simulink model "NavFilterTestHarness21"  (Simulink 7.9)
settings: Solver=FixedStepDiscrete  StartTime=min(IMUtime)  StopTime=max(IMUtime)  FixedStep=0.001  RelTol=1e-3
undefined symbols (not defined in the file or in its folder): accel, ADSframe, ADStime, angRate, ATTframe, CourseDeg, GndSpd, GPSframe, GPStime, Hgt, IMUframe, IMUtime, LatDeg, LngDeg, MagBiasX, MagBiasY, MagBiasZ, MAGframe, MAGtime, MagX, MagY, MagZ, Pitch, Roll, Veas, VelD, Yaw
libraries: simulink x13
(part 4 of 5)

== matlab function InertialNavFilter/Fuse True Airspeed Measurements ==
  data: states input double; P input double; FuseData input double; VtasMea input double; nextStates output double; nextP output double; innovation output double; StatesAtMeasTime input double; varInnov output double; useAirspeed input double
%#codegen
function [...
    nextStates, ... % state vector after fusion of measurements
    nextP, ... % state covariance matrix after fusion of corrections
    innovation, ... % True airspeed innovations (m/s)
    varInnov] ... % True airspeed innovation variance (m/s)^2
    = FuseAirspeed( ...
    states, ... % predicted states from the INS (q0, ... , q3, VelN,E,D, PosN,E,D, WindN,E, P0, camera roll pitch yaw misalignment)
    P, ... % predicted covariance
    FuseData, ... % Boolean to initiate fusion of airspeed measurements
    VtasMea, ... % true airspeed measurement (m/s)
    StatesAtMeasTime, ... % states at time of airspeed measurement
    useAirspeed) % Boolean to indicate that a airspeed sensor is being used

% initialise innovation
innovation = single(0);

% initialise innovation variance vector (for data analysis only)
varInnov = single(0);

% Airspeed measurement error variance (m/s)^2.
R_TAS = single(2.0);

% Copy required states to local variable names
vn = single(StatesAtMeasTime(5));
ve = single(StatesAtMeasTime(6));
vd = single(StatesAtMeasTime(7));
vwn = single(StatesAtMeasTime(14));
vwe = single(StatesAtMeasTime(15));

% define arrays used to calculate intermediate result in covariance
% update
KH  = single(zeros(21,21));
KHP = single(zeros(21,21));

% Calculate the airspeed prediction
VtasPred = sqrt((ve - vwe)^2 + (vn - vwn)^2 + vd^2);
% Need to check that it is flying before fusing airspeed data due to
if (useAirspeed && FuseData && (VtasPred > 1.0) && VtasMea > 8.0)
    % Sequential fusion of XYZ components
    
    % Calculate observation jacobians and Kalman gain
    SH_TAS = single(zeros(3,1));
    SH_TAS(1) = 1/((ve - vwe)^2 + (vn - vwn)^2 + vd^2)^(1/2);
    SH_TAS(2) = (SH_TAS(1)*(2*ve - 2*vwe))/2;
    SH_TAS(3) = (SH_TAS(1)*(2*vn - 2*vwn))/2;
    
    H_TAS = single(zeros(1,21));
    H_TAS(1,5) = SH_TAS(3);
    H_TAS(1,6) = SH_TAS(2);
    H_TAS(1,7) = vd*SH_TAS(1);
    H_TAS(1,14) = -SH_TAS(3);
    H_TAS(1,15) = -SH_TAS(2);
    
    SK_TAS = single(zeros(2,1));
    SK_TAS(1) = 1/(R_TAS + SH_TAS(3)*(P(5,5)*SH_TAS(3) + P(6,5)*SH_TAS(2) - P(14,5)*SH_TAS(3) - P(15,5)*SH_TAS(2) + P(7,5)*vd*SH_TAS(1)) + SH_TAS(2)*(P(5,6)*SH_TAS(3) + P(6,6)*SH_TAS(2) - P(14,6)*SH_TAS(3) - P(15,6)*SH_TAS(2) + P(7,6)*vd*SH_TAS(1)) - SH_TAS(3)*(P(5,14)*SH_TAS(3) + P(6,14)*SH_TAS(2) - P(14,14)*SH_TAS(3) - P(15,14)*SH_TAS(2) + P(7,14)*vd*SH_TAS(1)) - SH_TAS(2)*(P(5,15)*SH_TAS(3) + P(6,15)*SH_TAS(2) - P(14,15)*SH_TAS(3) - P(15,15)*SH_TAS(2) + P(7,15)*vd*SH_TAS(1)) + vd*SH_TAS(1)*(P(5,7)*SH_TAS(3) + P(6,7)*SH_TAS(2) - P(14,7)*SH_TAS(3) - P(15,7)*SH_TAS(2) + P(7,7)*vd*SH_TAS(1)));
    SK_TAS(2) = SH_TAS(2);
    
    K_TAS = single(zeros(21,1));
    K_TAS(1,1) = SK_TAS(1)*(P(1,5)*SH_TAS(3) - P(1,14)*SH_TAS(3) + P(1,6)*SK_TAS(2) - P(1,15)*SK_TAS(2) + P(1,7)*vd*SH_TAS(1));
    K_TAS(2,1) = SK_TAS(1)*(P(2,5)*SH_TAS(3) - P(2,14)*SH_TAS(3) + P(2,6)*SK_TAS(2) - P(2,15)*SK_TAS(2) + P(2,7)*vd*SH_TAS(1));
    K_TAS(3,1) = SK_TAS(1)*(P(3,5)*SH_TAS(3) - P(3,14)*SH_TAS(3) + P(3,6)*SK_TAS(2) - P(3,15)*SK_TAS(2) + P(3,7)*vd*SH_TAS(1));
    K_TAS(4,1) = SK_TAS(1)*(P(4,5)*SH_TAS(3) - P(4,14)*SH_TAS(3) + P(4,6)*SK_TAS(2) - P(4,15)*SK_TAS(2) + P(4,7)*vd*SH_TAS(1));
    K_TAS(5,1) = SK_TAS(1)*(P(5,5)*SH_TAS(3) - P(5,14)*SH_TAS(3) + P(5,6)*SK_TAS(2) - P(5,15)*SK_TAS(2) + P(5,7)*vd*SH_TAS(1));
    K_TAS(6,1) = SK_TAS(1)*(P(6,5)*SH_TAS(3) - P(6,14)*SH_TAS(3) + P(6,6)*SK_TAS(2) - P(6,15)*SK_TAS(2) + P(6,7)*vd*SH_TAS(1));
    K_TAS(7,1) = SK_TAS(1)*(P(7,5)*SH_TAS(3) - P(7,14)*SH_TAS(3) + P(7,6)*SK_TAS(2) - P(7,15)*SK_TAS(2) + P(7,7)*vd*SH_TAS(1));
    K_TAS(8,1) = SK_TAS(1)*(P(8,5)*SH_TAS(3) - P(8,14)*SH_TAS(3) + P(8,6)*SK_TAS(2) - P(8,15)*SK_TAS(2) + P(8,7)*vd*SH_TAS(1));
    K_TAS(9,1) = SK_TAS(1)*(P(9,5)*SH_TAS(3) - P(9,14)*SH_TAS(3) + P(9,6)*SK_TAS(2) - P(9,15)*SK_TAS(2) + P(9,7)*vd*SH_TAS(1));
    K_TAS(10,1) = SK_TAS(1)*(P(10,5)*SH_TAS(3) - P(10,14)*SH_TAS(3) + P(10,6)*SK_TAS(2) - P(10,15)*SK_TAS(2) + P(10,7)*vd*SH_TAS(1));
    K_TAS(11,1) = SK_TAS(1)*(P(11,5)*SH_TAS(3) - P(11,14)*SH_TAS(3) + P(11,6)*SK_TAS(2) - P(11,15)*SK_TAS(2) + P(11,7)*vd*SH_TAS(1));
    K_TAS(12,1) = SK_TAS(1)*(P(12,5)*SH_TAS(3) - P(12,14)*SH_TAS(3) + P(12,6)*SK_TAS(2) - P(12,15)*SK_TAS(2) + P(12,7)*vd*SH_TAS(1));
    K_TAS(13,1) = SK_TAS(1)*(P(13,5)*SH_TAS(3) - P(13,14)*SH_TAS(3) + P(13,6)*SK_TAS(2) - P(13,15)*SK_TAS(2) + P(13,7)*vd*SH_TAS(1));
    K_TAS(14,1) = SK_TAS(1)*(P(14,5)*SH_TAS(3) - P(14,14)*SH_TAS(3) + P(14,6)*SK_TAS(2) - P(14,15)*SK_TAS(2) + P(14,7)*vd*SH_TAS(1));
    K_TAS(15,1) = SK_TAS(1)*(P(15,5)*SH_TAS(3) - P(15,14)*SH_TAS(3) + P(15,6)*SK_TAS(2) - P(15,15)*SK_TAS(2) + P(15,7)*vd*SH_TAS(1));
    K_TAS(16,1) = SK_TAS(1)*(P(16,5)*SH_TAS(3) - P(16,14)*SH_TAS(3) + P(16,6)*SK_TAS(2) - P(16,15)*SK_TAS(2) + P(16,7)*vd*SH_TAS(1));
    K_TAS(17,1) = SK_TAS(1)*(P(17,5)*SH_TAS(3) - P(17,14)*SH_TAS(3) + P(17,6)*SK_TAS(2) - P(17,15)*SK_TAS(2) + P(17,7)*vd*SH_TAS(1));
    K_TAS(18,1) = SK_TAS(1)*(P(18,5)*SH_TAS(3) - P(18,14)*SH_TAS(3) + P(18,6)*SK_TAS(2) - P(18,15)*SK_TAS(2) + P(18,7)*vd*SH_TAS(1));
    K_TAS(19,1) = SK_TAS(1)*(P(19,5)*SH_TAS(3) - P(19,14)*SH_TAS(3) + P(19,6)*SK_TAS(2) - P(19,15)*SK_TAS(2) + P(19,7)*vd*SH_TAS(1));
    K_TAS(20,1) = SK_TAS(1)*(P(20,5)*SH_TAS(3) - P(20,14)*SH_TAS(3) + P(20,6)*SK_TAS(2) - P(20,15)*SK_TAS(2) + P(20,7)*vd*SH_TAS(1));
    K_TAS(21,1) = SK_TAS(1)*(P(21,5)*SH_TAS(3) - P(21,14)*SH_TAS(3) + P(21,6)*SK_TAS(2) - P(21,15)*SK_TAS(2) + P(21,7)*vd*SH_TAS(1));
    
    % calculate the innovation variance (for data logging only)
    varInnov = 1/SK_TAS(1);
    
    % Calculate the measurement innovation
    innovation = VtasPred - VtasMea;
    % Check the innovation for consistencey and don't fuse if > 5Sigma
    if (innovation*innovation*SK_TAS(1)) < 25.0
        xk = K_TAS * innovation;
        states = states - xk;
        % normalise the quaternion states
        quatMag = sqrt(states(1)^2 + states(2)^2 + states(3)^2 + states(4)^2);
        if (quatMag > 1e-12)
            states(1:4) = states(1:4) / quatMag;
        end
        % correct the covariance P = (I - K*H)*P
        % take advantage of the empty columns in H_TAS to reduce the
        % number of operations
        for i = 1:24
            for j = 5:7
                KH(i,j) = K_TAS(i)*H_TAS(j);
            end
            for j = 14:15
                KH(i,j) = K_TAS(i)*H_TAS(j);
            end
        end
        for i = 1:21
            for j = 1:21
                for k = 5:7
                    KHP(i,j) = KHP(i,j) + KH(i,k)*P(k,j);
                end
                for k = 14:15
                    KHP(i,j) = KHP(i,j) + KH(i,k)*P(k,j);
                end
            end
        end
        P = P - KHP;
        P = 0.5*(P + transpose(P));
    end
end

% Set default output for states and covariance
nextP = P;
nextStates   = states;

end

== matlab function InertialNavFilter/Store States at Magnetometer Meas Time ==
  data: FuseData output double; States input double; measDataArrived input double; StatesAtMeasTime output double; Ndelay input double; ratio input double
%#codegen
function [FuseData,StatesAtMeasTime]   = StoreStatesAtMeasTime(States,measDataArrived,Ndelay,ratio)

% Implement a state sampler that stores the state inoput from Ndelay 
% samples before the measurement is predicted to arrive. When the
% measurement arrives, the stored state is output along with a data fusion
% request. This enables the filter to account for lag in sensors that can
% in some cases be greater than 1 measurement time step. the delay time si
% specified in units of the state prediction delta time. For example if a 
% delay of 0.16 seconds was required, and the state prediction ran at 50 Hz
% then Ndelay would be set to 50*0.15 = 8.
% It is assumed that this function is called the same rate as the state 
% prediction, and that the measurement data comes in at a constant
% rate.
% The 'ratio'specifies the ratio of the state prediction to measurement
% data rates. For example if the state prediction occurres at 50Hz and the
% measurements are being received at 5Hz, then 'ratio' = 50/5 = 10

% This function avoids the need to use large data buffers
% It is generic function that can be used for states required by all
% measurement fusion processes, and as such has not been optimised to only
% includes the specific states required, or the buffer arry length trimmed
% to the minimum required.

% Ndelay cannot be zero and cannot exceed a value of 10*ratio-1
Ndelay = max(min(Ndelay,int32(10*ratio)),int32(1));

majorStepDelay = int32(ceil(single(Ndelay)/single(ratio)));
minorStepDelay = int32(rem(single(Ndelay),single(ratio)));

persistent prevStatesMatrix;
if isempty(prevStatesMatrix)
    prevStatesMatrix = single(zeros(21,11));
end

persistent totalFrameCount;
if isempty(totalFrameCount)
    totalFrameCount = int32(0);
end

persistent measID;
if isempty(measID)
    measID = int32(zeros(1,11));
end

persistent minorFrameCount;
if isempty(minorFrameCount)
    minorFrameCount = int32(0);
end

totalFrameCount = totalFrameCount + int32(1);
minorFrameCount = minorFrameCount + int32(1);

if measDataArrived
    if measID(1) ~= 0
        FuseData = logical(1);
    else
        FuseData = logical(0);
    end
    if abs(single(totalFrameCount - measID(1) - Ndelay)) < 0.5*single(ratio)
        StatesAtMeasTime = prevStatesMatrix(:,1);
    else
        frameErrors = abs(measID - totalFrameCount + Ndelay);
        bestError = Ndelay;
        bestIndex = int32(1);
        for index = 1:majorStepDelay
            if frameErrors(index) < bestError
                bestError = frameErrors(index);
                bestIndex = index;
            end
        end
        StatesAtMeasTime = prevStatesMatrix(:,bestIndex);
    end
else
    StatesAtMeasTime = single(zeros(21,1));
    FuseData = logical(0);
end

if minorFrameCount == (ratio - minorStepDelay)
    if majorStepDelay > int32(0)
        for index = 1:majorStepDelay
            prevStatesMatrix(:,index) = prevStatesMatrix(:,index+1);
            measID(index) = measID(index+1);
        end
    end
    prevStatesMatrix(:,majorStepDelay) = States;
    measID(majorStepDelay) = totalFrameCount;
end

if measDataArrived
    minorFrameCount = int32(0);
end

end

== matlab function InertialNavFilter/Calc Initial Parameters/Embedded MATLAB Function ==
  data: gravityNED output double; earthRateNED output double; covariance output double; latDeg input double
function [gravityNED, earthRateNED, covariance] = calculateInitialData(latDeg)
%#codegen

% degrees to to radians conversion
deg2rad = single(pi/180);

% Define the local gracity vector
gravityNED  = single([0;0;9.807]);

% Define the initial Euler angle covariance (Phi, Theta, Psi)
InitialEulerCovariance  = single([(1.0*pi/180); (1.0*pi/180); (10.0*pi/180)].^2);

% Define the transformation vector from a 321 sequence Euler rotation vector to a q0,...,q3 quaternion vector
% linearised around a level orientation (roll,pitch = 0,0)
J_eul2quat = ...
    single([[ 0.0, 0.0, 0.0]; ...
    [ 0.5, 0.0, 0.0]; ...
    [ 0.0, 0.5, 0.0]; ...
    [ 0.0, 0.0, 0.5]]);

% Form the covariance matrix for the intial Euler angle coordinates
angleCov = diag(InitialEulerCovariance);

% Transform the Euler angle covariances into the equivalent quaternion covariances
quatCov = J_eul2quat*angleCov*transpose(J_eul2quat);

% define the state covariances with the exception of the quaternion covariances
Sigma_vel_NE = single(0.7); % 1 sigma uncertainty in horizontal velocity components
Sigma_vel_D  = single(0.7); % 1 sigma uncertainty in vertical velocity
Sigma_pos_NE = single(15); % 1 sigma uncertainty in horizontal position components
Sigma_pos_D  = single(5.0); % 1 sigma uncertainty in vertical position
Sigma_dAng   = single(1/10*pi/180*0.02); % 1 Sigma uncertainty in delta angle bias
Sigma_wind   = single(8);
Sigma_MagNED = single(20);
Sigma_MagXYZ = single(20);
covariance   = single(diag([0;0;0;0;Sigma_vel_NE*[1;1];Sigma_vel_D;Sigma_pos_NE*[1;1];Sigma_pos_D;Sigma_dAng*[1;1;1];Sigma_wind*[1;1];Sigma_MagNED*[1;1;1];Sigma_MagXYZ*[1;1;1]].^2));

% Add the quaternion covariances
covariance(1:4,1:4) = quatCov;

%Define Earth rotation vector in the NED navigation frame
earthRateECEF = single([0; 0; 7.2921e-005]);
earthRateNED  = ...
    single([cos(latDeg*deg2rad)*earthRateECEF(3); ...
    0; ...
    -sin(latDeg*deg2rad)*earthRateECEF(3)]);

== matlab function InertialNavFilter/Store States at Height Meas Time ==
  data: FuseData output double; States input double; measDataArrived input double; StatesAtMeasTime output double; Ndelay input double; ratio input double
%#codegen
function [FuseData,StatesAtMeasTime]   = StoreStatesAtMeasTime(States,measDataArrived,Ndelay,ratio)

% Implement a state sampler that stores the state inoput from Ndelay 
% samples before the measurement is predicted to arrive. When the
% measurement arrives, the stored state is output along with a data fusion
% request. This enables the filter to account for lag in sensors that can
% in some cases be greater than 1 measurement time step. the delay time si
% specified in units of the state prediction delta time. For example if a 
% delay of 0.16 seconds was required, and the state prediction ran at 50 Hz
% then Ndelay would be set to 50*0.15 = 8.
% It is assumed that this function is called the same rate as the state 
% prediction, and that the measurement data comes in at a constant
% rate.
% The 'ratio'specifies the ratio of the state prediction to measurement
% data rates. For example if the state prediction occurres at 50Hz and the
% measurements are being received at 5Hz, then 'ratio' = 50/5 = 10

% This function avoids the need to use large data buffers
% It is generic function that can be used for states required by all
% measurement fusion processes, and as such has not been optimised to only
% includes the specific states required, or the buffer arry length trimmed
% to the minimum required.

% Ndelay cannot be zero and cannot exceed a value of 10*ratio-1
Ndelay = max(min(Ndelay,int32(10*ratio)),int32(1));

majorStepDelay = int32(ceil(single(Ndelay)/single(ratio)));
minorStepDelay = int32(rem(single(Ndelay),single(ratio)));

persistent prevStatesMatrix;
if isempty(prevStatesMatrix)
    prevStatesMatrix = single(zeros(21,11));
end

persistent totalFrameCount;
if isempty(totalFrameCount)
    totalFrameCount = int32(0);
end

persistent measID;
if isempty(measID)
    measID = int32(zeros(1,11));
end

persistent minorFrameCount;
if isempty(minorFrameCount)
    minorFrameCount = int32(0);
end

totalFrameCount = totalFrameCount + int32(1);
minorFrameCount = minorFrameCount + int32(1);

if measDataArrived
    if measID(1) ~= 0
        FuseData = logical(1);
    else
        FuseData = logical(0);
    end
    if abs(single(totalFrameCount - measID(1) - Ndelay)) < 0.5*single(ratio)
        StatesAtMeasTime = prevStatesMatrix(:,1);
    else
        frameErrors = abs(measID - totalFrameCount + Ndelay);
        bestError = Ndelay;
        bestIndex = int32(1);
        for index = 1:majorStepDelay
            if frameErrors(index) < bestError
                bestError = frameErrors(index);
                bestIndex = index;
            end
        end
        StatesAtMeasTime = prevStatesMatrix(:,bestIndex);
    end
else
    StatesAtMeasTime = single(zeros(21,1));
    FuseData = logical(0);
end

if minorFrameCount == (ratio - minorStepDelay)
    if majorStepDelay > int32(0)
        for index = 1:majorStepDelay
            prevStatesMatrix(:,index) = prevStatesMatrix(:,index+1);
            measID(index) = measID(index+1);
        end
    end
    prevStatesMatrix(:,majorStepDelay) = States;
    measID(majorStepDelay) = totalFrameCount;
end

if measDataArrived
    minorFrameCount = int32(0);
end

end

== matlab function InertialNavFilter/Store States at Vtas Meas Time ==
  data: FuseData output double; States input double; measDataArrived input double; StatesAtMeasTime output double; Ndelay input double; ratio input double
%#codegen
function [FuseData,StatesAtMeasTime]   = StoreStatesAtMeasTime(States,measDataArrived,Ndelay,ratio)

% Implement a state sampler that stores the state inoput from Ndelay 
% samples before the measurement is predicted to arrive. When the
% measurement arrives, the stored state is output along with a data fusion
% request. This enables the filter to account for lag in sensors that can
% in some cases be greater than 1 measurement time step. the delay time si
% specified in units of the state prediction delta time. For example if a 
% delay of 0.16 seconds was required, and the state prediction ran at 50 Hz
% then Ndelay would be set to 50*0.15 = 8.
% It is assumed that this function is called the same rate as the state 
% prediction, and that the measurement data comes in at a constant
% rate.
% The 'ratio'specifies the ratio of the state prediction to measurement
% data rates. For example if the state prediction occurres at 50Hz and the
% measurements are being received at 5Hz, then 'ratio' = 50/5 = 10

% This function avoids the need to use large data buffers
% It is generic function that can be used for states required by all
% measurement fusion processes, and as such has not been optimised to only
% includes the specific states required, or the buffer arry length trimmed
% to the minimum required.

% Ndelay cannot be zero and cannot exceed a value of 10*ratio-1
Ndelay = max(min(Ndelay,int32(10*ratio)),int32(1));

majorStepDelay = int32(ceil(single(Ndelay)/single(ratio)));
minorStepDelay = int32(rem(single(Ndelay),single(ratio)));

persistent prevStatesMatrix;
if isempty(prevStatesMatrix)
    prevStatesMatrix = single(zeros(21,11));
end

persistent totalFrameCount;
if isempty(totalFrameCount)
    totalFrameCount = int32(0);
end

persistent measID;
if isempty(measID)
    measID = int32(zeros(1,11));
end

persistent minorFrameCount;
if isempty(minorFrameCount)
    minorFrameCount = int32(0);
end

totalFrameCount = totalFrameCount + int32(1);
minorFrameCount = minorFrameCount + int32(1);

if measDataArrived
    if measID(1) ~= 0
        FuseData = logical(1);
    else
        FuseData = logical(0);
    end
    if abs(single(totalFrameCount - measID(1) - Ndelay)) < 0.5*single(ratio)
        StatesAtMeasTime = prevStatesMatrix(:,1);
    else
        frameErrors = abs(measID - totalFrameCount + Ndelay);
        bestError = Ndelay;
        bestIndex = int32(1);
        for index = 1:majorStepDelay
            if frameErrors(index) < bestError
                bestError = frameErrors(index);
                bestIndex = index;
            end
        end
        StatesAtMeasTime = prevStatesMatrix(:,bestIndex);
    end
else
    StatesAtMeasTime = single(zeros(21,1));
    FuseData = logical(0);
end

if minorFrameCount == (ratio - minorStepDelay)
    if majorStepDelay > int32(0)
        for index = 1:majorStepDelay
            prevStatesMatrix(:,index) = prevStatesMatrix(:,index+1);
            measID(index) = measID(index+1);
        end
    end
    prevStatesMatrix(:,majorStepDelay) = States;
    measID(majorStepDelay) = totalFrameCount;
end

if measDataArrived
    minorFrameCount = int32(0);
end

end

== matlab function InertialNavFilter/Fuse Magnetometer Measurements ==
  data: states input double; P input double; FuseData input double; MagData input double; StatesAtMeasTime input double; nextStates output double; nextP output double; innovation output double; varInnov output double; useCompass input double
%#codegen
function [...
    nextStates, ... % state vector after fusion of measurements
    nextP, ... % state covariance matrix after fusion of corrections
    innovation, ... % Magnetometer innovations - milligauss
    varInnov] ... % Innovation variances - millgauss^2
    = FuseMagnetometer( ...
    states, ... % predicted states
    P, ... % predicted covariance
    FuseData, ... % Boolean to initiate fusion of magnetometer measurements
    MagData, ... % Magnetic flux measurements (milliGauss)
    StatesAtMeasTime, ... % states at time of airspeed measurement
    useCompass) % Boolean to indicate that a Magnetometer is being used

persistent q0 q1 q2 q3 magN magE magD;
if isempty(q0)
    q0 = single(1);
end
if isempty(q1)
    q1 = single(0);
end
if isempty(q2)
    q2 = single(0);
end
if isempty(q3)
    q3 = single(0);
end
if isempty(magN)
    magN = single(0);
end
if isempty(magE)
    magE = single(0);
end
if isempty(magD)
    magD = single(0);
end
persistent obsIndex
if isempty(obsIndex)
    obsIndex = 1;
end
persistent SH_MAG
if isempty(SH_MAG)
    SH_MAG = single(zeros(9,1));
end
persistent Tnb
if isempty(Tnb)
    Tnb = single(eye(3,3));
end
persistent MagPred
if isempty(MagPred)
    MagPred = single(zeros(3,1));
end

% declare array used to calculate intermediate result in covariance
% update
KH  = single(zeros(21,21));
KHP = single(zeros(21,21));

% define magnetometer measurement error variance (milligauss).
R_MAG = single(50^2);

% declare innovation variances
varInnov = single(zeros(3,1));

% declare innovation vector
innovation = single(zeros(1,3));

% Perform sequential fusion of Magnetometer measurements.
% This assumes that the errors in the dfferent componenets are
% uncorrelated which is not true, however in the absence of covariance
% data fit is the only assumption we can make
% so we might as well take advantage of the computational efficiencies
% associated with sequential fusion
if (useCompass && FuseData) || (useCompass && (obsIndex == 2 || obsIndex == 3))
    % Sequential fusion of XYZ components to spread processing load across
    % three prediction time steps.
    % Calculate observation jacobians and Kalman gains
    K_MAG = single(zeros(21,1));
    H_MAG = single(zeros(1,21));
    if FuseData
        % Copy required states to local variable names
        q0 = StatesAtMeasTime(1);
        q1 = StatesAtMeasTime(2);
        q2 = StatesAtMeasTime(3);
        q3 = StatesAtMeasTime(4);
        magN = StatesAtMeasTime(16);
        magE = StatesAtMeasTime(17);
        magD = StatesAtMeasTime(18);
        % rotate predicted earth components into body axes and calculate
        % predicted measurments
        Tnb = single([q0^2 + q1^2 - q2^2 - q3^2, 2*(q1*q2 + q0*q3) , 2*(q1*q3-q0*q2) ;...
            2*(q1*q2 - q0*q3), q0^2 - q1^2 + q2^2 - q3^2, 2*(q2*q3 + q0*q1);...
            2*(q1*q3 + q0*q2) , 2*(q2*q3 - q0*q1) , q0^2 - q1^2 - q2^2 + q3^2]);
        MagPred = Tnb*StatesAtMeasTime(16:18) + StatesAtMeasTime(19:21);
        % Calculate observation jacobian common terms
        SH_MAG(1) = 2*magD*q3 + 2*magE*q2 + 2*magN*q1;
        SH_MAG(2) = 2*magD*q0 - 2*magE*q1 + 2*magN*q2;
        SH_MAG(3) = 2*magD*q1 + 2*magE*q0 - 2*magN*q3;
        SH_MAG(4) = q3^2;
        SH_MAG(5) = q2^2;
        SH_MAG(6) = q1^2;
        SH_MAG(7) = q0^2;
        SH_MAG(8) = 2*magN*q0;
        SH_MAG(9) = 2*magE*q3;
        % calculate observation jacobian
        H_MAG = single(zeros(1,21));
        H_MAG(1,1) = SH_MAG(8) + SH_MAG(9) - 2*magD*q2;
        H_MAG(1,2) = SH_MAG(1);
        H_MAG(1,3) = 2*magE*q1 - 2*magD*q0 - 2*magN*q2;
        H_MAG(1,4) = SH_MAG(3);
        H_MAG(1,16) = SH_MAG(6) - SH_MAG(5) - SH_MAG(4) + SH_MAG(7);
        H_MAG(1,17) = 2*q0*q3 + 2*q1*q2;
        H_MAG(1,18) = 2*q1*q3 - 2*q0*q2;
        H_MAG(1,19) = 1;
        % calculate Kalman gain
        SK_MX = zeros(6,1);
        SK_MX(1) = 1/(P(19,19) + R_MAG + P(2,19)*SH_MAG(1) + P(4,19)*SH_MAG(3) - P(16,19)*(SH_MAG(4) + SH_MAG(5) - SH_MAG(6) - SH_MAG(7)) - (2*magD*q0 - 2*magE*q1 + 2*magN*q2)*(P(19,3) + P(2,3)*SH_MAG(1) + P(4,3)*SH_MAG(3) - P(16,3)*(SH_MAG(4) + SH_MAG(5) - SH_MAG(6) - SH_MAG(7)) + P(17,3)*(2*q0*q3 + 2*q1*q2) - P(18,3)*(2*q0*q2 - 2*q1*q3) - P(3,3)*(2*magD*q0 - 2*magE*q1 + 2*magN*q2) + P(1,3)*(SH_MAG(8) + SH_MAG(9) - 2*magD*q2)) + (SH_MAG(8) + SH_MAG(9) - 2*magD*q2)*(P(19,1) + P(2,1)*SH_MAG(1) + P(4,1)*SH_MAG(3) - P(16,1)*(SH_MAG(4) + SH_MAG(5) - SH_MAG(6) - SH_MAG(7)) + P(17,1)*(2*q0*q3 + 2*q1*q2) - P(18,1)*(2*q0*q2 - 2*q1*q3) - P(3,1)*(2*magD*q0 - 2*magE*q1 + 2*magN*q2) + P(1,1)*(SH_MAG(8) + SH_MAG(9) - 2*magD*q2)) + SH_MAG(1)*(P(19,2) + P(2,2)*SH_MAG(1) + P(4,2)*SH_MAG(3) - P(16,2)*(SH_MAG(4) + SH_MAG(5) - SH_MAG(6) - SH_MAG(7)) + P(17,2)*(2*q0*q3 + 2*q1*q2) - P(18,2)*(2*q0*q2 - 2*q1*q3) - P(3,2)*(2*magD*q0 - 2*magE*q1 + 2*magN*q2) + P(1,2)*(SH_MAG(8) + SH_MAG(9) - 2*magD*q2)) + SH_MAG(3)*(P(19,4) + P(2,4)*SH_MAG(1) + P(4,4)*SH_MAG(3) - P(16,4)*(SH_MAG(4) + SH_MAG(5) - SH_MAG(6) - SH_MAG(7)) + P(17,4)*(2*q0*q3 + 2*q1*q2) - P(18,4)*(2*q0*q2 - 2*q1*q3) - P(3,4)*(2*magD*q0 - 2*magE*q1 + 2*magN*q2) + P(1,4)*(SH_MAG(8) + SH_MAG(9) - 2*magD*q2)) - (SH_MAG(4) + SH_MAG(5) - SH_MAG(6) - SH_MAG(7))*(P(19,16) + P(2,16)*SH_MAG(1) + P(4,16)*SH_MAG(3) - P(16,16)*(SH_MAG(4) + SH_MAG(5) - SH_MAG(6) - SH_MAG(7)) + P(17,16)*(2*q0*q3 + 2*q1*q2) - P(18,16)*(2*q0*q2 - 2*q1*q3) - P(3,16)*(2*magD*q0 - 2*magE*q1 + 2*magN*q2) + P(1,16)*(SH_MAG(8) + SH_MAG(9) - 2*magD*q2)) + P(17,19)*(2*q0*q3 + 2*q1*q2) - P(18,19)*(2*q0*q2 - 2*q1*q3) - P(3,19)*(2*magD*q0 - 2*magE*q1 + 2*magN*q2) + (2*q0*q3 + 2*q1*q2)*(P(19,17) + P(2,17)*SH_MAG(1) + P(4,17)*SH_MAG(3) - P(16,17)*(SH_MAG(4) + SH_MAG(5) - SH_MAG(6) - SH_MAG(7)) + P(17,17)*(2*q0*q3 + 2*q1*q2) - P(18,17)*(2*q0*q2 - 2*q1*q3) - P(3,17)*(2*magD*q0 - 2*magE*q1 + 2*magN*q2) + P(1,17)*(SH_MAG(8) + SH_MAG(9) - 2*magD*q2)) - (2*q0*q2 - 2*q1*q3)*(P(19,18) + P(2,18)*SH_MAG(1) + P(4,18)*SH_MAG(3) - P(16,18)*(SH_MAG(4) + SH_MAG(5) - SH_MAG(6) - SH_MAG(7)) + P(17,18)*(2*q0*q3 + 2*q1*q2) - P(18,18)*(2*q0*q2 - 2*q1*q3) - P(3,18)*(2*magD*q0 - 2*magE*q1 + 2*magN*q2) + P(1,18)*(SH_MAG(8) + SH_MAG(9) - 2*magD*q2)) + P(1,19)*(SH_MAG(8) + SH_MAG(9) - 2*magD*q2));
        SK_MX(2) = SH_MAG(4) + SH_MAG(5) - SH_MAG(6) - SH_MAG(7);
        SK_MX(3) = 2*magD*q0 - 2*magE*q1 + 2*magN*q2;
        SK_MX(4) = SH_MAG(8) + SH_MAG(9) - 2*magD*q2;
        SK_MX(5) = 2*q0*q2 - 2*q1*q3;
        SK_MX(6) = 2*q0*q3 + 2*q1*q2;
        K_MAG = single(zeros(21,1));
        K_MAG(1,1) = SK_MX(1)*(P(1,19) + P(1,2)*SH_MAG(1) + P(1,4)*SH_MAG(3) + P(1,1)*SK_MX(4) - P(1,3)*SK_MX(3) - P(1,16)*SK_MX(2) + P(1,17)*SK_MX(6) - P(1,18)*SK_MX(5));
        K_MAG(2,1) = SK_MX(1)*(P(2,19) + P(2,2)*SH_MAG(1) + P(2,4)*SH_MAG(3) + P(2,1)*SK_MX(4) - P(2,3)*SK_MX(3) - P(2,16)*SK_MX(2) + P(2,17)*SK_MX(6) - P(2,18)*SK_MX(5));
        K_MAG(3,1) = SK_MX(1)*(P(3,19) + P(3,2)*SH_MAG(1) + P(3,4)*SH_MAG(3) + P(3,1)*SK_MX(4) - P(3,3)*SK_MX(3) - P(3,16)*SK_MX(2) + P(3,17)*SK_MX(6) - P(3,18)*SK_MX(5));
        K_MAG(4,1) = SK_MX(1)*(P(4,19) + P(4,2)*SH_MAG(1) + P(4,4)*SH_MAG(3) + P(4,1)*SK_MX(4) - P(4,3)*SK_MX(3) - P(4,16)*SK_MX(2) + P(4,17)*SK_MX(6) - P(4,18)*SK_MX(5));
        K_MAG(5,1) = SK_MX(1)*(P(5,19) + P(5,2)*SH_MAG(1) + P(5,4)*SH_MAG(3) + P(5,1)*SK_MX(4) - P(5,3)*SK_MX(3) - P(5,16)*SK_MX(2) + P(5,17)*SK_MX(6) - P(5,18)*SK_MX(5));
        K_MAG(6,1) = SK_MX(1)*(P(6,19) + P(6,2)*SH_MAG(1) + P(6,4)*SH_MAG(3) + P(6,1)*SK_MX(4) - P(6,3)*SK_MX(3) - P(6,16)*SK_MX(2) + P(6,17)*SK_MX(6) - P(6,18)*SK_MX(5));
        K_MAG(7,1) = SK_MX(1)*(P(7,19) + P(7,2)*SH_MAG(1) + P(7,4)*SH_MAG(3) + P(7,1)*SK_MX(4) - P(7,3)*SK_MX(3) - P(7,16)*SK_MX(2) + P(7,17)*SK_MX(6) - P(7,18)*SK_MX(5));
        K_MAG(8,1) = SK_MX(1)*(P(8,19) + P(8,2)*SH_MAG(1) + P(8,4)*SH_MAG(3) + P(8,1)*SK_MX(4) - P(8,3)*SK_MX(3) - P(8,16)*SK_MX(2) + P(8,17)*SK_MX(6) - P(8,18)*SK_MX(5));
        K_MAG(9,1) = SK_MX(1)*(P(9,19) + P(9,2)*SH_MAG(1) + P(9,4)*SH_MAG(3) + P(9,1)*SK_MX(4) - P(9,3)*SK_MX(3) - P(9,16)*SK_MX(2) + P(9,17)*SK_MX(6) - P(9,18)*SK_MX(5));
        K_MAG(10,1) = SK_MX(1)*(P(10,19) + P(10,2)*SH_MAG(1) + P(10,4)*SH_MAG(3) + P(10,1)*SK_MX(4) - P(10,3)*SK_MX(3) - P(10,16)*SK_MX(2) + P(10,17)*SK_MX(6) - P(10,18)*SK_MX(5));
        K_MAG(11,1) = SK_MX(1)*(P(11,19) + P(11,2)*SH_MAG(1) + P(11,4)*SH_MAG(3) + P(11,1)*SK_MX(4) - P(11,3)*SK_MX(3) - P(11,16)*SK_MX(2) + P(11,17)*SK_MX(6) - P(11,18)*SK_MX(5));
        K_MAG(12,1) = SK_MX(1)*(P(12,19) + P(12,2)*SH_MAG(1) + P(12,4)*SH_MAG(3) + P(12,1)*SK_MX(4) - P(12,3)*SK_MX(3) - P(12,16)*SK_MX(2) + P(12,17)*SK_MX(6) - P(12,18)*SK_MX(5));
        K_MAG(13,1) = SK_MX(1)*(P(13,19) + P(13,2)*SH_MAG(1) + P(13,4)*SH_MAG(3) + P(13,1)*SK_MX(4) - P(13,3)*SK_MX(3) - P(13,16)*SK_MX(2) + P(13,17)*SK_MX(6) - P(13,18)*SK_MX(5));
        K_MAG(14,1) = SK_MX(1)*(P(14,19) + P(14,2)*SH_MAG(1) + P(14,4)*SH_MAG(3) + P(14,1)*SK_MX(4) - P(14,3)*SK_MX(3) - P(14,16)*SK_MX(2) + P(14,17)*SK_MX(6) - P(14,18)*SK_MX(5));
        K_MAG(15,1) = SK_MX(1)*(P(15,19) + P(15,2)*SH_MAG(1) + P(15,4)*SH_MAG(3) + P(15,1)*SK_MX(4) - P(15,3)*SK_MX(3) - P(15,16)*SK_MX(2) + P(15,17)*SK_MX(6) - P(15,18)*SK_MX(5));
        K_MAG(16,1) = SK_MX(1)*(P(16,19) + P(16,2)*SH_MAG(1) + P(16,4)*SH_MAG(3) + P(16,1)*SK_MX(4) - P(16,3)*SK_MX(3) - P(16,16)*SK_MX(2) + P(16,17)*SK_MX(6) - P(16,18)*SK_MX(5));
        K_MAG(17,1) = SK_MX(1)*(P(17,19) + P(17,2)*SH_MAG(1) + P(17,4)*SH_MAG(3) + P(17,1)*SK_MX(4) - P(17,3)*SK_MX(3) - P(17,16)*SK_MX(2) + P(17,17)*SK_MX(6) - P(17,18)*SK_MX(5));
        K_MAG(18,1) = SK_MX(1)*(P(18,19) + P(18,2)*SH_MAG(1) + P(18,4)*SH_MAG(3) + P(18,1)*SK_MX(4) - P(18,3)*SK_MX(3) - P(18,16)*SK_MX(2) + P(18,17)*SK_MX(6) - P(18,18)*SK_MX(5));
        K_MAG(19,1) = SK_MX(1)*(P(19,19) + P(19,2)*SH_MAG(1) + P(19,4)*SH_MAG(3) + P(19,1)*SK_MX(4) - P(19,3)*SK_MX(3) - P(19,16)*SK_MX(2) + P(19,17)*SK_MX(6) - P(19,18)*SK_MX(5));
        K_MAG(20,1) = SK_MX(1)*(P(20,19) + P(20,2)*SH_MAG(1) + P(20,4)*SH_MAG(3) + P(20,1)*SK_MX(4) - P(20,3)*SK_MX(3) - P(20,16)*SK_MX(2) + P(20,17)*SK_MX(6) - P(20,18)*SK_MX(5));
        K_MAG(21,1) = SK_MX(1)*(P(21,19) + P(21,2)*SH_MAG(1) + P(21,4)*SH_MAG(3) + P(21,1)*SK_MX(4) - P(21,3)*SK_MX(3) - P(21,16)*SK_MX(2) + P(21,17)*SK_MX(6) - P(21,18)*SK_MX(5));
        varInnov(1) = 1/SK_MX(1);
        % reset the observation index to 1 (we start by fusing the X
        % measurement)
        obsIndex = 1;
    elseif obsIndex == 2 % we are now fusing the Y measurement
        H_MAG = single(zeros(1,21));
        H_MAG(1,1) = SH_MAG(3);
        H_MAG(1,2) = SH_MAG(2);
        H_MAG(1,3) = SH_MAG(1);
        H_MAG(1,4) = 2*magD*q2 - SH_MAG(9) - SH_MAG(8);
        H_MAG(1,16) = 2*q1*q2 - 2*q0*q3;
        H_MAG(1,17) = SH_MAG(5) - SH_MAG(4) - SH_MAG(6) + SH_MAG(7);
        H_MAG(1,18) = 2*q0*q1 + 2*q2*q3;
        H_MAG(1,20) = 1;
        % calculate the Kalman gain
        SK_MY = single(zeros(5,1));
        SK_MY(1) = 1/(P(20,20) + R_MAG + P(1,20)*SH_MAG(3) + P(2,20)*SH_MAG(2) + P(3,20)*SH_MAG(1) - P(17,20)*(SH_MAG(4) - SH_MAG(5) + SH_MAG(6) - SH_MAG(7)) - (2*q0*q3 - 2*q1*q2)*(P(20,16) + P(1,16)*SH_MAG(3) + P(2,16)*SH_MAG(2) + P(3,16)*SH_MAG(1) - P(17,16)*(SH_MAG(4) - SH_MAG(5) + SH_MAG(6) - SH_MAG(7)) - P(16,16)*(2*q0*q3 - 2*q1*q2) + P(18,16)*(2*q0*q1 + 2*q2*q3) - P(4,16)*(SH_MAG(8) + SH_MAG(9) - 2*magD*q2)) + (2*q0*q1 + 2*q2*q3)*(P(20,18) + P(1,18)*SH_MAG(3) + P(2,18)*SH_MAG(2) + P(3,18)*SH_MAG(1) - P(17,18)*(SH_MAG(4) - SH_MAG(5) + SH_MAG(6) - SH_MAG(7)) - P(16,18)*(2*q0*q3 - 2*q1*q2) + P(18,18)*(2*q0*q1 + 2*q2*q3) - P(4,18)*(SH_MAG(8) + SH_MAG(9) - 2*magD*q2)) - (SH_MAG(8) + SH_MAG(9) - 2*magD*q2)*(P(20,4) + P(1,4)*SH_MAG(3) + P(2,4)*SH_MAG(2) + P(3,4)*SH_MAG(1) - P(17,4)*(SH_MAG(4) - SH_MAG(5) + SH_MAG(6) - SH_MAG(7)) - P(16,4)*(2*q0*q3 - 2*q1*q2) + P(18,4)*(2*q0*q1 + 2*q2*q3) - P(4,4)*(SH_MAG(8) + SH_MAG(9) - 2*magD*q2)) - P(16,20)*(2*q0*q3 - 2*q1*q2) + P(18,20)*(2*q0*q1 + 2*q2*q3) + SH_MAG(3)*(P(20,1) + P(1,1)*SH_MAG(3) + P(2,1)*SH_MAG(2) + P(3,1)*SH_MAG(1) - P(17,1)*(SH_MAG(4) - SH_MAG(5) + SH_MAG(6) - SH_MAG(7)) - P(16,1)*(2*q0*q3 - 2*q1*q2) + P(18,1)*(2*q0*q1 + 2*q2*q3) - P(4,1)*(SH_MAG(8) + SH_MAG(9) - 2*magD*q2)) + SH_MAG(2)*(P(20,2) + P(1,2)*SH_MAG(3) + P(2,2)*SH_MAG(2) + P(3,2)*SH_MAG(1) - P(17,2)*(SH_MAG(4) - SH_MAG(5) + SH_MAG(6) - SH_MAG(7)) - P(16,2)*(2*q0*q3 - 2*q1*q2) + P(18,2)*(2*q0*q1 + 2*q2*q3) - P(4,2)*(SH_MAG(8) + SH_MAG(9) - 2*magD*q2)) + SH_MAG(1)*(P(20,3) + P(1,3)*SH_MAG(3) + P(2,3)*SH_MAG(2) + P(3,3)*SH_MAG(1) - P(17,3)*(SH_MAG(4) - SH_MAG(5) + SH_MAG(6) - SH_MAG(7)) - P(16,3)*(2*q0*q3 - 2*q1*q2) + P(18,3)*(2*q0*q1 + 2*q2*q3) - P(4,3)*(SH_MAG(8) + SH_MAG(9) - 2*magD*q2)) - (SH_MAG(4) - SH_MAG(5) + SH_MAG(6) - SH_MAG(7))*(P(20,17) + P(1,17)*SH_MAG(3) + P(2,17)*SH_MAG(2) + P(3,17)*SH_MAG(1) - P(17,17)*(SH_MAG(4) - SH_MAG(5) + SH_MAG(6) - SH_MAG(7)) - P(16,17)*(2*q0*q3 - 2*q1*q2) + P(18,17)*(2*q0*q1 + 2*q2*q3) - P(4,17)*(SH_MAG(8) + SH_MAG(9) - 2*magD*q2)) - P(4,20)*(SH_MAG(8) + SH_MAG(9) - 2*magD*q2));
        SK_MY(2) = SH_MAG(4) - SH_MAG(5) + SH_MAG(6) - SH_MAG(7);
        SK_MY(3) = SH_MAG(8) + SH_MAG(9) - 2*magD*q2;
        SK_MY(4) = 2*q0*q3 - 2*q1*q2;
        SK_MY(5) = 2*q0*q1 + 2*q2*q3;
        K_MAG = single(zeros(21,1));
        K_MAG(1,1) = SK_MY(1)*(P(1,20) + P(1,1)*SH_MAG(3) + P(1,2)*SH_MAG(2) + P(1,3)*SH_MAG(1) - P(1,4)*SK_MY(3) - P(1,17)*SK_MY(2) - P(1,16)*SK_MY(4) + P(1,18)*SK_MY(5));
        K_MAG(2,1) = SK_MY(1)*(P(2,20) + P(2,1)*SH_MAG(3) + P(2,2)*SH_MAG(2) + P(2,3)*SH_MAG(1) - P(2,4)*SK_MY(3) - P(2,17)*SK_MY(2) - P(2,16)*SK_MY(4) + P(2,18)*SK_MY(5));
        K_MAG(3,1) = SK_MY(1)*(P(3,20) + P(3,1)*SH_MAG(3) + P(3,2)*SH_MAG(2) + P(3,3)*SH_MAG(1) - P(3,4)*SK_MY(3) - P(3,17)*SK_MY(2) - P(3,16)*SK_MY(4) + P(3,18)*SK_MY(5));
        K_MAG(4,1) = SK_MY(1)*(P(4,20) + P(4,1)*SH_MAG(3) + P(4,2)*SH_MAG(2) + P(4,3)*SH_MAG(1) - P(4,4)*SK_MY(3) - P(4,17)*SK_MY(2) - P(4,16)*SK_MY(4) + P(4,18)*SK_MY(5));
        K_MAG(5,1) = SK_MY(1)*(P(5,20) + P(5,1)*SH_MAG(3) + P(5,2)*SH_MAG(2) + P(5,3)*SH_MAG(1) - P(5,4)*SK_MY(3) - P(5,17)*SK_MY(2) - P(5,16)*SK_MY(4) + P(5,18)*SK_MY(5));
        K_MAG(6,1) = SK_MY(1)*(P(6,20) + P(6,1)*SH_MAG(3) + P(6,2)*SH_MAG(2) + P(6,3)*SH_MAG(1) - P(6,4)*SK_MY(3) - P(6,17)*SK_MY(2) - P(6,16)*SK_MY(4) + P(6,18)*SK_MY(5));
        K_MAG(7,1) = SK_MY(1)*(P(7,20) + P(7,1)*SH_MAG(3) + P(7,2)*SH_MAG(2) + P(7,3)*SH_MAG(1) - P(7,4)*SK_MY(3) - P(7,17)*SK_MY(2) - P(7,16)*SK_MY(4) + P(7,18)*SK_MY(5));
        K_MAG(8,1) = SK_MY(1)*(P(8,20) + P(8,1)*SH_MAG(3) + P(8,2)*SH_MAG(2) + P(8,3)*SH_MAG(1) - P(8,4)*SK_MY(3) - P(8,17)*SK_MY(2) - P(8,16)*SK_MY(4) + P(8,18)*SK_MY(5));
        K_MAG(9,1) = SK_MY(1)*(P(9,20) + P(9,1)*SH_MAG(3) + P(9,2)*SH_MAG(2) + P(9,3)*SH_MAG(1) - P(9,4)*SK_MY(3) - P(9,17)*SK_MY(2) - P(9,16)*SK_MY(4) + P(9,18)*SK_MY(5));
        K_MAG(10,1) = SK_MY(1)*(P(10,20) + P(10,1)*SH_MAG(3) + P(10,2)*SH_MAG(2) + P(10,3)*SH_MAG(1) - P(10,4)*SK_MY(3) - P(10,17)*SK_MY(2) - P(10,16)*SK_MY(4) + P(10,18)*SK_MY(5));
        K_MAG(11,1) = SK_MY(1)*(P(11,20) + P(11,1)*SH_MAG(3) + P(11,2)*SH_MAG(2) + P(11,3)*SH_MAG(1) - P(11,4)*SK_MY(3) - P(11,17)*SK_MY(2) - P(11,16)*SK_MY(4) + P(11,18)*SK_MY(5));
        K_MAG(12,1) = SK_MY(1)*(P(12,20) + P(12,1)*SH_MAG(3) + P(12,2)*SH_MAG(2) + P(12,3)*SH_MAG(1) - P(12,4)*SK_MY(3) - P(12,17)*SK_MY(2) - P(12,16)*SK_MY(4) + P(12,18)*SK_MY(5));
        K_MAG(13,1) = SK_MY(1)*(P(13,20) + P(13,1)*SH_MAG(3) + P(13,2)*SH_MAG(2) + P(13,3)*SH_MAG(1) - P(13,4)*SK_MY(3) - P(13,17)*SK_MY(2) - P(13,16)*SK_MY(4) + P(13,18)*SK_MY(5));
        K_MAG(14,1) = SK_MY(1)*(P(14,20) + P(14,1)*SH_MAG(3) + P(14,2)*SH_MAG(2) + P(14,3)*SH_MAG(1) - P(14,4)*SK_MY(3) - P(14,17)*SK_MY(2) - P(14,16)*SK_MY(4) + P(14,18)*SK_MY(5));
        K_MAG(15,1) = SK_MY(1)*(P(15,20) + P(15,1)*SH_MAG(3) + P(15,2)*SH_MAG(2) + P(15,3)*SH_MAG(1) - P(15,4)*SK_MY(3) - P(15,17)*SK_MY(2) - P(15,16)*SK_MY(4) + P(15,18)*SK_MY(5));
        K_MAG(16,1) = SK_MY(1)*(P(16,20) + P(16,1)*SH_MAG(3) + P(16,2)*SH_MAG(2) + P(16,3)*SH_MAG(1) - P(16,4)*SK_MY(3) - P(16,17)*SK_MY(2) - P(16,16)*SK_MY(4) + P(16,18)*SK_MY(5));
        K_MAG(17,1) = SK_MY(1)*(P(17,20) + P(17,1)*SH_MAG(3) + P(17,2)*SH_MAG(2) + P(17,3)*SH_MAG(1) - P(17,4)*SK_MY(3) - P(17,17)*SK_MY(2) - P(17,16)*SK_MY(4) + P(17,18)*SK_MY(5));
        K_MAG(18,1) = SK_MY(1)*(P(18,20) + P(18,1)*SH_MAG(3) + P(18,2)*SH_MAG(2) + P(18,3)*SH_MAG(1) - P(18,4)*SK_MY(3) - P(18,17)*SK_MY(2) - P(18,16)*SK_MY(4) + P(18,18)*SK_MY(5));
        K_MAG(19,1) = SK_MY(1)*(P(19,20) + P(19,1)*SH_MAG(3) + P(19,2)*SH_MAG(2) + P(19,3)*SH_MAG(1) - P(19,4)*SK_MY(3) - P(19,17)*SK_MY(2) - P(19,16)*SK_MY(4) + P(19,18)*SK_MY(5));
        K_MAG(20,1) = SK_MY(1)*(P(20,20) + P(20,1)*SH_MAG(3) + P(20,2)*SH_MAG(2) + P(20,3)*SH_MAG(1) - P(20,4)*SK_MY(3) - P(20,17)*SK_MY(2) - P(20,16)*SK_MY(4) + P(20,18)*SK_MY(5));
        K_MAG(21,1) = SK_MY(1)*(P(21,20) + P(21,1)*SH_MAG(3) + P(21,2)*SH_MAG(2) + P(21,3)*SH_MAG(1) - P(21,4)*SK_MY(3) - P(21,17)*SK_MY(2) - P(21,16)*SK_MY(4) + P(21,18)*SK_MY(5));
        varInnov(2) = 1/SK_MY(1);
    elseif obsIndex == 3 % we are now fusing the Z measurement
        % calculate the observation jacobian
        H_MAG = single(zeros(1,21));
        H_MAG(1,1) = SH_MAG(2);
        H_MAG(1,2) = 2*magN*q3 - 2*magE*q0 - 2*magD*q1;
        H_MAG(1,3) = SH_MAG(8) + SH_MAG(9) - 2*magD*q2;
        H_MAG(1,4) = SH_MAG(1);
        H_MAG(1,16) = 2*q0*q2 + 2*q1*q3;
        H_MAG(1,17) = 2*q2*q3 - 2*q0*q1;
        H_MAG(1,18) = SH_MAG(4) - SH_MAG(5) - SH_MAG(6) + SH_MAG(7);
        H_MAG(1,21) = 1;
        % calculate the Kalman gain
        SK_MZ = zeros(6,1);
        SK_MZ(1) = 1/(P(21,21) + R_MAG + P(1,21)*SH_MAG(2) + P(4,21)*SH_MAG(1) + P(18,21)*(SH_MAG(4) - SH_MAG(5) - SH_MAG(6) + SH_MAG(7)) - (2*magD*q1 + 2*magE*q0 - 2*magN*q3)*(P(21,2) + P(1,2)*SH_MAG(2) + P(4,2)*SH_MAG(1) + P(18,2)*(SH_MAG(4) - SH_MAG(5) - SH_MAG(6) + SH_MAG(7)) + P(16,2)*(2*q0*q2 + 2*q1*q3) - P(17,2)*(2*q0*q1 - 2*q2*q3) - P(2,2)*(2*magD*q1 + 2*magE*q0 - 2*magN*q3) + P(3,2)*(SH_MAG(8) + SH_MAG(9) - 2*magD*q2)) + (SH_MAG(8) + SH_MAG(9) - 2*magD*q2)*(P(21,3) + P(1,3)*SH_MAG(2) + P(4,3)*SH_MAG(1) + P(18,3)*(SH_MAG(4) - SH_MAG(5) - SH_MAG(6) + SH_MAG(7)) + P(16,3)*(2*q0*q2 + 2*q1*q3) - P(17,3)*(2*q0*q1 - 2*q2*q3) - P(2,3)*(2*magD*q1 + 2*magE*q0 - 2*magN*q3) + P(3,3)*(SH_MAG(8) + SH_MAG(9) - 2*magD*q2)) + SH_MAG(2)*(P(21,1) + P(1,1)*SH_MAG(2) + P(4,1)*SH_MAG(1) + P(18,1)*(SH_MAG(4) - SH_MAG(5) - SH_MAG(6) + SH_MAG(7)) + P(16,1)*(2*q0*q2 + 2*q1*q3) - P(17,1)*(2*q0*q1 - 2*q2*q3) - P(2,1)*(2*magD*q1 + 2*magE*q0 - 2*magN*q3) + P(3,1)*(SH_MAG(8) + SH_MAG(9) - 2*magD*q2)) + SH_MAG(1)*(P(21,4) + P(1,4)*SH_MAG(2) + P(4,4)*SH_MAG(1) + P(18,4)*(SH_MAG(4) - SH_MAG(5) - SH_MAG(6) + SH_MAG(7)) + P(16,4)*(2*q0*q2 + 2*q1*q3) - P(17,4)*(2*q0*q1 - 2*q2*q3) - P(2,4)*(2*magD*q1 + 2*magE*q0 - 2*magN*q3) + P(3,4)*(SH_MAG(8) + SH_MAG(9) - 2*magD*q2)) + (SH_MAG(4) - SH_MAG(5) - SH_MAG(6) + SH_MAG(7))*(P(21,18) + P(1,18)*SH_MAG(2) + P(4,18)*SH_MAG(1) + P(18,18)*(SH_MAG(4) - SH_MAG(5) - SH_MAG(6) + SH_MAG(7)) + P(16,18)*(2*q0*q2 + 2*q1*q3) - P(17,18)*(2*q0*q1 - 2*q2*q3) - P(2,18)*(2*magD*q1 + 2*magE*q0 - 2*magN*q3) + P(3,18)*(SH_MAG(8) + SH_MAG(9) - 2*magD*q2)) + P(16,21)*(2*q0*q2 + 2*q1*q3) - P(17,21)*(2*q0*q1 - 2*q2*q3) - P(2,21)*(2*magD*q1 + 2*magE*q0 - 2*magN*q3) + (2*q0*q2 + 2*q1*q3)*(P(21,16) + P(1,16)*SH_MAG(2) + P(4,16)*SH_MAG(1) + P(18,16)*(SH_MAG(4) - SH_MAG(5) - SH_MAG(6) + SH_MAG(7)) + P(16,16)*(2*q0*q2 + 2*q1*q3) - P(17,16)*(2*q0*q1 - 2*q2*q3) - P(2,16)*(2*magD*q1 + 2*magE*q0 - 2*magN*q3) + P(3,16)*(SH_MAG(8) + SH_MAG(9) - 2*magD*q2)) - (2*q0*q1 - 2*q2*q3)*(P(21,17) + P(1,17)*SH_MAG(2) + P(4,17)*SH_MAG(1) + P(18,17)*(SH_MAG(4) - SH_MAG(5) - SH_MAG(6) + SH_MAG(7)) + P(16,17)*(2*q0*q2 + 2*q1*q3) - P(17,17)*(2*q0*q1 - 2*q2*q3) - P(2,17)*(2*magD*q1 + 2*magE*q0 - 2*magN*q3) + P(3,17)*(SH_MAG(8) + SH_MAG(9) - 2*magD*q2)) + P(3,21)*(SH_MAG(8) + SH_MAG(9) - 2*magD*q2));
        SK_MZ(2) = SH_MAG(4) - SH_MAG(5) - SH_MAG(6) + SH_MAG(7);
        SK_MZ(3) = 2*magD*q1 + 2*magE*q0 - 2*magN*q3;
        SK_MZ(4) = SH_MAG(8) + SH_MAG(9) - 2*magD*q2;
        SK_MZ(5) = 2*q0*q1 - 2*q2*q3;
        SK_MZ(6) = 2*q0*q2 + 2*q1*q3;
        K_MAG = single(zeros(21,1));
        K_MAG(1,1) = SK_MZ(1)*(P(1,21) + P(1,1)*SH_MAG(2) + P(1,4)*SH_MAG(1) - P(1,2)*SK_MZ(3) + P(1,3)*SK_MZ(4) + P(1,18)*SK_MZ(2) + P(1,16)*SK_MZ(6) - P(1,17)*SK_MZ(5));
        K_MAG(2,1) = SK_MZ(1)*(P(2,21) + P(2,1)*SH_MAG(2) + P(2,4)*SH_MAG(1) - P(2,2)*SK_MZ(3) + P(2,3)*SK_MZ(4) + P(2,18)*SK_MZ(2) + P(2,16)*SK_MZ(6) - P(2,17)*SK_MZ(5));
        K_MAG(3,1) = SK_MZ(1)*(P(3,21) + P(3,1)*SH_MAG(2) + P(3,4)*SH_MAG(1) - P(3,2)*SK_MZ(3) + P(3,3)*SK_MZ(4) + P(3,18)*SK_MZ(2) + P(3,16)*SK_MZ(6) - P(3,17)*SK_MZ(5));
        K_MAG(4,1) = SK_MZ(1)*(P(4,21) + P(4,1)*SH_MAG(2) + P(4,4)*SH_MAG(1) - P(4,2)*SK_MZ(3) + P(4,3)*SK_MZ(4) + P(4,18)*SK_MZ(2) + P(4,16)*SK_MZ(6) - P(4,17)*SK_MZ(5));
        K_MAG(5,1) = SK_MZ(1)*(P(5,21) + P(5,1)*SH_MAG(2) + P(5,4)*SH_MAG(1) - P(5,2)*SK_MZ(3) + P(5,3)*SK_MZ(4) + P(5,18)*SK_MZ(2) + P(5,16)*SK_MZ(6) - P(5,17)*SK_MZ(5));
        K_MAG(6,1) = SK_MZ(1)*(P(6,21) + P(6,1)*SH_MAG(2) + P(6,4)*SH_MAG(1) - P(6,2)*SK_MZ(3) + P(6,3)*SK_MZ(4) + P(6,18)*SK_MZ(2) + P(6,16)*SK_MZ(6) - P(6,17)*SK_MZ(5));
        K_MAG(7,1) = SK_MZ(1)*(P(7,21) + P(7,1)*SH_MAG(2) + P(7,4)*SH_MAG(1) - P(7,2)*SK_MZ(3) + P(7,3)*SK_MZ(4) + P(7,18)*SK_MZ(2) + P(7,16)*SK_MZ(6) - P(7,17)*SK_MZ(5));
        K_MAG(8,1) = SK_MZ(1)*(P(8,21) + P(8,1)*SH_MAG(2) + P(8,4)*SH_MAG(1) - P(8,2)*SK_MZ(3) + P(8,3)*SK_MZ(4) + P(8,18)*SK_MZ(2) + P(8,16)*SK_MZ(6) - P(8,17)*SK_MZ(5));
        K_MAG(9,1) = SK_MZ(1)*(P(9,21) + P(9,1)*SH_MAG(2) + P(9,4)*SH_MAG(1) - P(9,2)*SK_MZ(3) + P(9,3)*SK_MZ(4) + P(9,18)*SK_MZ(2) + P(9,16)*SK_MZ(6) - P(9,17)*SK_MZ(5));
        K_MAG(10,1) = SK_MZ(1)*(P(10,21) + P(10,1)*SH_MAG(2) + P(10,4)*SH_MAG(1) - P(10,2)*SK_MZ(3) + P(10,3)*SK_MZ(4) + P(10,18)*SK_MZ(2) + P(10,16)*SK_MZ(6) - P(10,17)*SK_MZ(5));
        K_MAG(11,1) = SK_MZ(1)*(P(11,21) + P(11,1)*SH_MAG(2) + P(11,4)*SH_MAG(1) - P(11,2)*SK_MZ(3) + P(11,3)*SK_MZ(4) + P(11,18)*SK_MZ(2) + P(11,16)*SK_MZ(6) - P(11,17)*SK_MZ(5));
        K_MAG(12,1) = SK_MZ(1)*(P(12,21) + P(12,1)*SH_MAG(2) + P(12,4)*SH_MAG(1) - P(12,2)*SK_MZ(3) + P(12,3)*SK_MZ(4) + P(12,18)*SK_MZ(2) + P(12,16)*SK_MZ(6) - P(12,17)*SK_MZ(5));
        K_MAG(13,1) = SK_MZ(1)*(P(13,21) + P(13,1)*SH_MAG(2) + P(13,4)*SH_MAG(1) - P(13,2)*SK_MZ(3) + P(13,3)*SK_MZ(4) + P(13,18)*SK_MZ(2) + P(13,16)*SK_MZ(6) - P(13,17)*SK_MZ(5));
        K_MAG(14,1) = SK_MZ(1)*(P(14,21) + P(14,1)*SH_MAG(2) + P(14,4)*SH_MAG(1) - P(14,2)*SK_MZ(3) + P(14,3)*SK_MZ(4) + P(14,18)*SK_MZ(2) + P(14,16)*SK_MZ(6) - P(14,17)*SK_MZ(5));
        K_MAG(15,1) = SK_MZ(1)*(P(15,21) + P(15,1)*SH_MAG(2) + P(15,4)*SH_MAG(1) - P(15,2)*SK_MZ(3) + P(15,3)*SK_MZ(4) + P(15,18)*SK_MZ(2) + P(15,16)*SK_MZ(6) - P(15,17)*SK_MZ(5));
        K_MAG(16,1) = SK_MZ(1)*(P(16,21) + P(16,1)*SH_MAG(2) + P(16,4)*SH_MAG(1) - P(16,2)*SK_MZ(3) + P(16,3)*SK_MZ(4) + P(16,18)*SK_MZ(2) + P(16,16)*SK_MZ(6) - P(16,17)*SK_MZ(5));
        K_MAG(17,1) = SK_MZ(1)*(P(17,21) + P(17,1)*SH_MAG(2) + P(17,4)*SH_MAG(1) - P(17,2)*SK_MZ(3) + P(17,3)*SK_MZ(4) + P(17,18)*SK_MZ(2) + P(17,16)*SK_MZ(6) - P(17,17)*SK_MZ(5));
        K_MAG(18,1) = SK_MZ(1)*(P(18,21) + P(18,1)*SH_MAG(2) + P(18,4)*SH_MAG(1) - P(18,2)*SK_MZ(3) + P(18,3)*SK_MZ(4) + P(18,18)*SK_MZ(2) + P(18,16)*SK_MZ(6) - P(18,17)*SK_MZ(5));
        K_MAG(19,1) = SK_MZ(1)*(P(19,21) + P(19,1)*SH_MAG(2) + P(19,4)*SH_MAG(1) - P(19,2)*SK_MZ(3) + P(19,3)*SK_MZ(4) + P(19,18)*SK_MZ(2) + P(19,16)*SK_MZ(6) - P(19,17)*SK_MZ(5));
        K_MAG(20,1) = SK_MZ(1)*(P(20,21) + P(20,1)*SH_MAG(2) + P(20,4)*SH_MAG(1) - P(20,2)*SK_MZ(3) + P(20,3)*SK_MZ(4) + P(20,18)*SK_MZ(2) + P(20,16)*SK_MZ(6) - P(20,17)*SK_MZ(5));
        K_MAG(21,1) = SK_MZ(1)*(P(21,21) + P(21,1)*SH_MAG(2) + P(21,4)*SH_MAG(1) - P(21,2)*SK_MZ(3) + P(21,3)*SK_MZ(4) + P(21,18)*SK_MZ(2) + P(21,16)*SK_MZ(6) - P(21,17)*SK_MZ(5));
        varInnov(3) = 1/SK_MZ(1);
    end
    % Calculate the measurement innovation
    innovation(obsIndex) = MagPred(obsIndex) - MagData(obsIndex);
    % Check the innovation for consistencey and don't fuse if > 5Sigma
    if ((innovation(obsIndex)^2) / varInnov(obsIndex)) < 25.0
        xk = K_MAG * innovation(obsIndex);
        states = states - xk;
        % normalise the quaternion states
        quatMag = sqrt(states(1)^2 + states(2)^2 + states(3)^2 + states(4)^2);
        if (quatMag > 1e-12)
            states(1:4) = states(1:4) / quatMag;
        end
        % correct the covariance P = (I - K*H)*P
        % take advantage of the empty columns in H_MAG to reduce the
        % number of operations
        for i = 1:24
            for j = 1:4
                KH(i,j) = K_MAG(i)*H_MAG(j);
            end
            for j = 16:21
                KH(i,j) = K_MAG(i)*H_MAG(j);
            end
        end
        for i = 1:21
            for j = 1:21
                for k = 1:4
                    KHP(i,j) = KHP(i,j) + KH(i,k)*P(k,j);
                end
                for k = 16:21
                    KHP(i,j) = KHP(i,j) + KH(i,k)*P(k,j);
                end
            end
        end
        P = P - KHP;
    end
    obsIndex = obsIndex + 1;
end
% Force symmetry on the covariance matrix to prevent ill-conditioning
% of the matrix which would cause the filter to blow-up
P = 0.5*(P + transpose(P));
% Set default output for states and covariance
nextP = P;
nextStates = states;
end

== matlab function LogData/Embedded MATLAB Function ==
  data: eulVar output double; states input double; quatCov input double
%#codegen
function eulVar  = calcEulerVariances(states,quatCov)

eulVar = zeros(1,3);

q0 = states(1);
q1 = states(2);
q2 = states(3);
q3 = states(4);

SJ = zeros(5,1);
SJ(1) = 1/(((2*q0*q3 + 2*q1*q2)/q0^2 + q1^2 - q2^2 - q3^2)^2 + 1);
SJ(2) = 1/(((2*q0*q1 + 2*q2*q3)/q0^2 - q1^2 - q2^2 + q3^2)^2 + 1);
SJ(3) = 1/(1 - (2*q0*q2 - 2*q1*q3)^2)^(1/2);
SJ(4) = 1/q0^2;
SJ(5) = 1/q0^3;

J = zeros(3,4);
J(1,1) = SJ(2)*(2*q1*SJ(4) - 2*SJ(5)*(2*q0*q1 + 2*q2*q3));
J(1,2) = -SJ(2)*(2*q1 - 2/q0);
J(1,3) = -SJ(2)*(2*q2 - 2*q3*SJ(4));
J(1,4) = SJ(2)*(2*q3 + 2*q2*SJ(4));
J(2,1) = 2*q2*SJ(3);
J(2,2) = -2*q3*SJ(3);
J(2,3) = 2*q0*SJ(3);
J(2,4) = -2*q1*SJ(3);
J(3,1) = SJ(1)*(2*q3*SJ(4) - 2*SJ(5)*(2*q0*q3 + 2*q1*q2));
J(3,2) = SJ(1)*(2*q1 + 2*q2*SJ(4));
J(3,3) = -SJ(1)*(2*q2 - 2*q1*SJ(4));
J(3,4) = -SJ(1)*(2*q3 - 2/q0);

% Transform the Euler angle covariances into the equivalent quaternion covariances
eulCov = J*quatCov*transpose(J);

eulVar(1) = eulCov(1,1);
eulVar(2) = eulCov(2,2);
eulVar(3) = eulCov(3,3);


return

== matlab function LogData/Convert GPS Data ==
  data: LatLongDeg input double; GndSpd input double; CourseDeg input double; VelD input double; VelNED output double; PosNE output double; RefLatLongDeg input double
%#codegen
function [VelNED,PosNE]   = ConvertGpsData(LatLongDeg,GndSpd,CourseDeg,VelD,RefLatLongDeg)

% Do a conversion from lat,long to local North.Est position relative to a
% reference point using WGS-84 eaerth radius and using a simple spherical
% earth model
% Convert GPS course and speed to North and East velocity components

deg2rad = single(pi/180);
earthRadius = single(6378145);

PosNE = single(zeros(2,1));
VelNED = single(zeros(3,1));
LatLongDelta = (LatLongDeg-RefLatLongDeg) * deg2rad;
PosNE(1) = earthRadius * LatLongDelta(1);
PosNE(2) = earthRadius * cos(RefLatLongDeg(1)*deg2rad) * LatLongDelta(2);
VelNED(1) = GndSpd*cos(CourseDeg*deg2rad);
VelNED(2) = GndSpd*sin(CourseDeg*deg2rad);
VelNED(3) = VelD;

return
